simulink model "surge_model_linear"  (R2014a)
settings: Solver=ode45  StartTime=tstart  StopTime=tstop  RelTol=1e-3
values from neighbouring files (symbols this model uses):
  nc = 80*2*pi/60    (= 8.37758040957)    [run_task_1_6.m]
undefined symbols (not defined in the file or in its folder): K, T
settings Model: Creator=Hwk  LastModifiedBy=Hwk

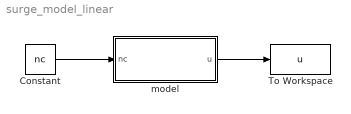
== system surge_model_linear ==
  Constant : Constant  Value=nc
  To Workspace : ToWorkspace  VariableName=u  SampleTime=10
  model : Subsystem
  wires:
  model/1(u) -> To Workspace/1
  Constant/1 -> model/1(nc)

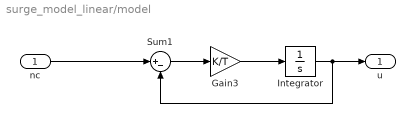
== system surge_model_linear/model ==
  nc : Inport
  Gain3 : Gain  Gain=K/T
  Integrator : Integrator
  Sum1 : Sum  Inputs=|+-
  u : Outport
  wires:
  Integrator/1 -> Sum1/2, u/1
  nc/1 -> Sum1/1
  Sum1/1 -> Gain3/1
  Gain3/1 -> Integrator/1
